simulink model "testmodel"  (R2017b)
settings: Solver=FixedStepAuto  StartTime=0.0  StopTime=inf  FixedStep=.001  RelTol=1e-3  EnableMultiTasking=on
libraries: simulink x5, dspstat3 x5
settings Model: SimulationMode=external  Creator=MRRL  LastModifiedBy=johnm_000
settings SolverCC: PositivePriorityOrder=on
settings OptimizationCC: PassReuseOutputArgsThreshold=0  MaxStackSize=64
settings DebuggingCC: ParameterTunabilityLossMsg=error
settings HardwareCC: ProdBitPerPointer=32  ProdBitPerSizeT=32  ProdBitPerPtrDiffT=32  ProdLargestAtomicInteger=Long  ProdLargestAtomicFloat=Double  ProdWordSize=32  ProdHWDeviceType=ARM Compatible->ARM Cortex  UseEmbeddedCoderFeatures=off  UseSimulinkCoderFeatures=off
settings SFSimCC: MATLABDynamicMemAlloc=off
settings RTWCC: SystemTargetFile=ert.tlc  HardwareBoard=Raspberry Pi  TemplateMakefile=ert_default_tmf  GenerateReport=on  Toolchain=GNU GCC Raspberry Pi  LaunchReport=on
settings CodeAppCC: ForceParamTrailComments=on  OperatorAnnotations=on
settings ERTTargetCC: ERTCustomFileBanners=off  SupportContinuousTime=on  SupportNonInlinedSFcns=on  RemoveResetFunc=off  SupportVariableSizeSignals=on  ModelStepFunctionPrototypeControlCompliant=off

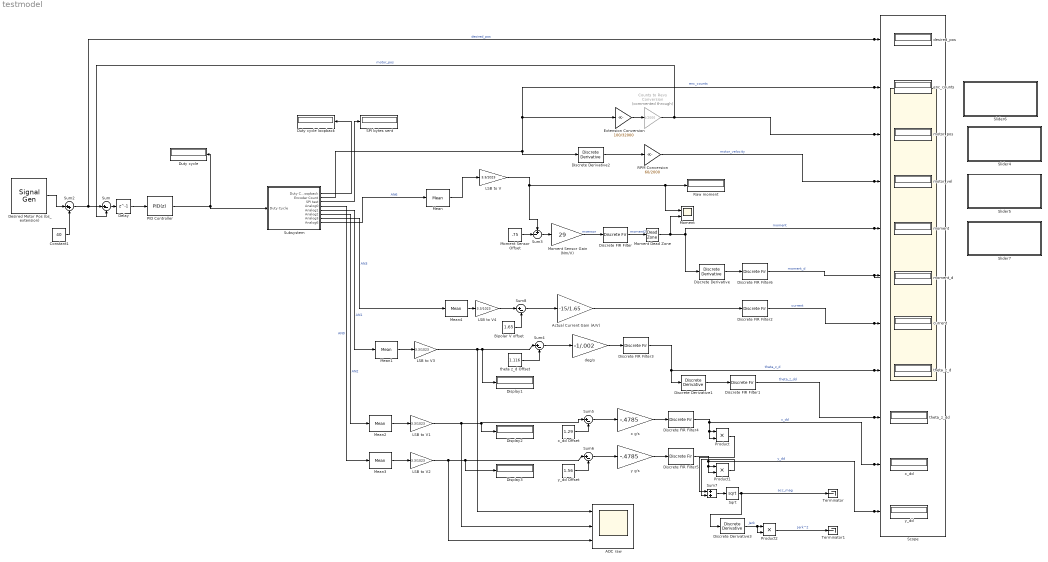
== system testmodel ==
  ADC raw : Scope  NumInputPorts=3
  Actual Current Gain (A/V) : Gain  Gain=-15/1.65
  Bipolar V offset : Constant  Value=1.65
  Constant1 : Constant  Value=40
  Counts to Revs Conversion : Gain  Commented=through  Gain=1/2000  ParamDataTypeStr=double  OutDataTypeStr=double
  Delay : Delay  DelayLength=1  InitialCondition=0
  Desired Motor Pos (bs_extension) : SignalGenerator  WaveForm=square  Amplitude=40
  Discrete Derivative{,1..3} (4 alike) : simulink/Discrete/Discrete Derivative  gainval=1.0  ICPrevScaledInput=0.0  InputProcessing=Inherited  OutMin=[]  OutMax=[]  OutDataType=fixdt(1, 16)  OutScaling=2^-10  DoSatur=off
  Discrete FIR Filter{,1..6} (7 alike) : DiscreteFir  Coefficients=[.1 .1 .1 .1 .1 .1 .1 .1 .1 .1]
  Display1 : Display
  Display2 : Display
  Display3 : Display
  Duty cycle : Display
  Duty cycle loopback : Display
  Extension Conversion : Gain  Gain=100/32000  ParamDataTypeStr=double  OutDataTypeStr=double
  LSB to V{,1..4} (5 alike) : Gain  Gain=3.3/1023
  Mean{,1..4} (5 alike) : dspstat3/Mean  run=off  reset_popup=None  InputProcessing=Columns as channels (frame based)  directionMode=Each column  dimension=1  roiEnable=off  roiType=Rectangles  roiPortion=Entire ROI  roiOutput=Individual statistics for each ROI  roiFlag=off  outputDataTypeStr=Inherit: Same as accumulator  outputLastDataTypeStr=Inherit: Same as accumulator  outputMin=[]  outputMax=[]  roundingMode=Floor  overflowMode=off
  Moment : Scope  NumInputPorts=2
  Moment Sensor Offset : Constant  Value=.75
  Moment Dead Zone : DeadZone  LowerValue=-.25  UpperValue=.25  SaturateOnIntegerOverflow=on
  Moment Sensor Gain (Nm/V) : Gain  Gain=29
  PID Controller : simulink/Continuous/PID Controller  Controller=PID  TimeDomain=Discrete-time  SampleTime=-1  IntegratorMethod=Forward Euler  FilterMethod=Forward Euler  Form=Parallel  UseFilter=on  ControllerParametersSource=internal  P=.1  I=.05  D=.003  N=300  InitialConditionSource=internal  InitialConditionForIntegrator=0  InitialConditionForFilter=0  ExternalReset=none  LimitOutput=on  UpperSaturationLimit=10  LowerSaturationLimit=-10  LinearizeAsGain=on  AntiWindupMode=none  Kb=1  TrackingMode=off  Kt=1  PParamMin=[]  PParamMax=[]  IParamMin=[]  IParamMax=[]  DParamMin=[]  DParamMax=[]  NParamMin=[]  NParamMax=[]  KbParamMin=[]  KbParamMax=[]  KtParamMin=[]  KtParamMax=[]  POutMin=[]  POutMax=[]  IOutMin=[]  IOutMax=[]  DOutMin=[]  DOutMax=[]  NOutMin=[]  NOutMax=[]  KbOutMin=[]  KbOutMax=[]  KtOutMin=[]  KtOutMax=[]  IntegratorOutMin=[]  IntegratorOutMax=[]  FilterOutMin=[]  FilterOutMax=[]  SumOutMin=[]  SumOutMax=[]  SumI1OutMin=[]  SumI1OutMax=[]  SumI2OutMin=[]  SumI2OutMax=[]  SumI3OutMin=[]  SumI3OutMax=[]  SumDOutMin=[]  SumDOutMax=[]  SaturationOutMin=[]  SaturationOutMax=[]  IntegratorContinuousStateAttributes=''  IntegratorStateMustResolveToSignalObject=off  IntegratorRTWStateStorageClass=Auto  FilterContinuousStateAttributes=''  FilterStateMustResolveToSignalObject=off  FilterRTWStateStorageClass=Auto  DifferentiatorICPrevScaledInput=0  DifferentiatorOutMin=[]  DifferentiatorOutMax=[]  InitialConditionSetting=State (most efficient)  FilterDiffOutCoefMin=[]  FilterDiffOutCoefMax=[]  SumDenOutMin=[]  SumDenOutMax=[]  SumNumOutMin=[]  SumNumOutMax=[]  ReciprocalOutMin=[]  ReciprocalOutMax=[]  DivideOutMin=[]  DivideOutMax=[]  TunerSelectOption=Transfer Function Based (PID Tuner App)
  Product : Product
  Product1 : Product
  Product2 : Product
  RPM Conversion : Gain  Gain=60/2000  ParamDataTypeStr=double  OutDataTypeStr=double
  Raw moment : Display
  SPI bytes sent : Display
  Scope : Scope  NumInputPorts=11
  Slider4 : Subsystem  DialogController=hmiCreateDDGDialog  IsWebBlock=on  mask(MWDashboardBlock){webBlockId=085e5637-d5ac-41cb-8731-7366e30fa1b6, webBlockType=slider, ShowInLibBrowser=on, ShowInitialText=on, HMISrcModelName=testmodel}
      mask prompts: webBlockId "WebBlock Id"; webBlockType "WebBlock Type"; HMISrcModelName "Source Model"
      mask Help: helpview([docroot '/mapfiles/simulink.map'], 'hmi_slider')
      mask Display:
      | if strcmp(get_param(bdroot(gcb),'BlockDiagramType'), 'library')
      |     image([(matlabroot) '/toolbox/simulink/hmi/icons/Slider.png']);
      | end
  Slider5 : Subsystem  DialogController=hmiCreateDDGDialog  IsWebBlock=on  mask(MWDashboardBlock){webBlockId=f28c714c-6520-4032-bd51-1fb2bc96d9d9, webBlockType=slider, ShowInLibBrowser=on, ShowInitialText=on, HMISrcModelName=testmodel}
      mask prompts: webBlockId "WebBlock Id"; webBlockType "WebBlock Type"; HMISrcModelName "Source Model"
      mask Help: helpview([docroot '/mapfiles/simulink.map'], 'hmi_slider')
      mask Display:
      | if strcmp(get_param(bdroot(gcb),'BlockDiagramType'), 'library')
      |     image([(matlabroot) '/toolbox/simulink/hmi/icons/Slider.png']);
      | end
  Slider6 : Subsystem  DialogController=hmiCreateDDGDialog  IsWebBlock=on  mask(MWDashboardBlock){webBlockId=46740757-b30e-4b65-9acf-b82be8f8e4ac, webBlockType=slider, ShowInLibBrowser=on, ShowInitialText=on, HMISrcModelName=testmodel}
      mask prompts: webBlockId "WebBlock Id"; webBlockType "WebBlock Type"; HMISrcModelName "Source Model"
      mask Help: helpview([docroot '/mapfiles/simulink.map'], 'hmi_slider')
      mask Display:
      | if strcmp(get_param(bdroot(gcb),'BlockDiagramType'), 'library')
      |     image([(matlabroot) '/toolbox/simulink/hmi/icons/Slider.png']);
      | end
  Slider7 : Subsystem  DialogController=hmiCreateDDGDialog  IsWebBlock=on  mask(MWDashboardBlock){webBlockId=fcfba7e5-e6d5-4b75-8ef5-2454024f1223, webBlockType=slider, ShowInLibBrowser=on, ShowInitialText=on, HMISrcModelName=testmodel}
      mask prompts: webBlockId "WebBlock Id"; webBlockType "WebBlock Type"; HMISrcModelName "Source Model"
      mask Help: helpview([docroot '/mapfiles/simulink.map'], 'hmi_slider')
      mask Display:
      | if strcmp(get_param(bdroot(gcb),'BlockDiagramType'), 'library')
      |     image([(matlabroot) '/toolbox/simulink/hmi/icons/Slider.png']);
      | end
  Sqrt : Sqrt  SaturateOnIntegerOverflow=on
  Subsystem : Subsystem
  Sum{,4..6,8} (5 alike) : Sum  Inputs=|+-
  Sum2 : Sum  Inputs=|++
  Sum3 : Sum  Inputs=+-|
  Sum7 : Sum
  Terminator : Terminator
  Terminator1 : Terminator
  current : Display
  deg/s : Gain  Gain=-1/.002
  desired_pos : Display
  enc_counts : Display
  moment : Display
  moment_d : Display
  motor_pos : Display
  motor_vel : Display
  "theta z_d Offset " : Constant  Value=1.116
  theta_z_d : Display
  theta_z_dd : Display
  x g's : Gain  Gain=-.4785
  x_dd : Display
  x_dd Offset : Constant  Value=1.29
  y g's : Gain  Gain=-.4785
  y_dd : Display
  y_dd Offset : Constant  Value=1.56
  wires:
  LSB to V4/1 -> Sum8/1
  Sum2/1 -> desired_pos/1, Scope/1, Sum/1  "desired_pos"
  Subsystem/2(Encoder Count) -> enc_counts/1, Scope/2, Extension Conversion/1, Discrete Derivative2/1  "enc_counts"
  Discrete FIR Filter6/1 -> moment_d/1, Scope/6  "moment_d"
  Extension Conversion/1 -> Counts to Revs Conversion/1
  Mean4/1 -> LSB to V4/1
  Discrete Derivative/1 -> Discrete FIR Filter6/1
  Discrete FIR Filter/1 -> Moment Dead Zone/1  "moment2"
  PID Controller/1 -> Subsystem/1(Duty Cycle), Duty cycle/1
  Subsystem/7(Analog3) -> Mean4/1  "AN3"
  LSB to V1/1 -> ADC raw/2, Display2/1, Sum5/1
  Subsystem/4(Analog0) -> Mean3/1  "AN0"
  Desired Motor Pos (bs_extension)/1 -> Sum2/1
  x_dd Offset/1 -> Sum5/2
  Counts to Revs Conversion/1 -> motor_pos/1, Scope/3, Sum/2  "motor_pos"
  Constant1/1 -> Sum2/2
  Subsystem/3(SPI test) -> SPI bytes sent/1
  RPM Conversion/1 -> motor_vel/1, Scope/4  "motor_velocity"
  Mean3/1 -> LSB to V2/1
  Bipolar V offset/1 -> Sum8/2
  LSB to V/1 -> Sum3/1, Raw moment/1, Moment/1
  Moment Dead Zone/1 -> moment/1, Scope/5, Discrete Derivative/1, Moment/2  "moment"
  Sum7/1 -> Sqrt/1
  Mean/1 -> LSB to V/1
  Product/1 -> Sum7/1
  Moment Sensor Offset/1 -> Sum3/2
  Discrete Derivative2/1 -> RPM Conversion/1
  Product1/1 -> Sum7/2
  Product2/1 -> Terminator1/1  "Jerk^2"
  Discrete FIR Filter5/1 -> y_dd/1, Scope/11, Product1/2, Product1/1  "y_dd"
  Moment Sensor Gain (Nm/V)/1 -> Discrete FIR Filter/1  "msensor"
  x g's/1 -> Discrete FIR Filter4/1
  Discrete FIR Filter4/1 -> x_dd/1, Scope/10, Product/2, Product/1  "x_dd"
  Actual Current Gain (A/V)/1 -> Discrete FIR Filter2/1
  y g's/1 -> Discrete FIR Filter5/1
  Discrete Derivative3/1 -> Product2/2, Product2/1  "Jerk"
  Sum6/1 -> y g's/1
  Subsystem/1(Duty Cycle Loopback) -> Duty cycle loopback/1
  Subsystem/8(Analog6) -> Mean/1  "AN6"
  y_dd Offset/1 -> Sum6/2
  Discrete FIR Filter1/1 -> theta_z_dd/1, Scope/9  "theta_z_dd"
  Mean1/1 -> LSB to V3/1
  Sqrt/1 -> Terminator/1, Discrete Derivative3/1  "acc_mag"
  Sum8/1 -> Actual Current Gain (A/V)/1
  LSB to V2/1 -> ADC raw/3, Display3/1, Sum6/1
  Sum5/1 -> x g's/1
  "theta z_d Offset "/1 -> Sum4/2
  Subsystem/5(Analog1) -> Mean1/1  "AN1"
  Delay/1 -> PID Controller/1
  LSB to V3/1 -> ADC raw/1, Display1/1, Sum4/1
  Subsystem/6(Analog2) -> Mean2/1  "AN2"
  Sum4/1 -> deg/s/1
  Discrete FIR Filter3/1 -> theta_z_d/1, Scope/8, Discrete Derivative1/1  "theta_z_d"
  Sum3/1 -> Moment Sensor Gain (Nm/V)/1
  Discrete FIR Filter2/1 -> current/1, Scope/7  "current"
  Discrete Derivative1/1 -> Discrete FIR Filter1/1
  Sum/1 -> Delay/1
  deg/s/1 -> Discrete FIR Filter3/1
  Mean2/1 -> LSB to V1/1

== system testmodel/Slider4 ==

== system testmodel/Slider5 ==

== system testmodel/Slider6 ==

== system testmodel/Slider7 ==

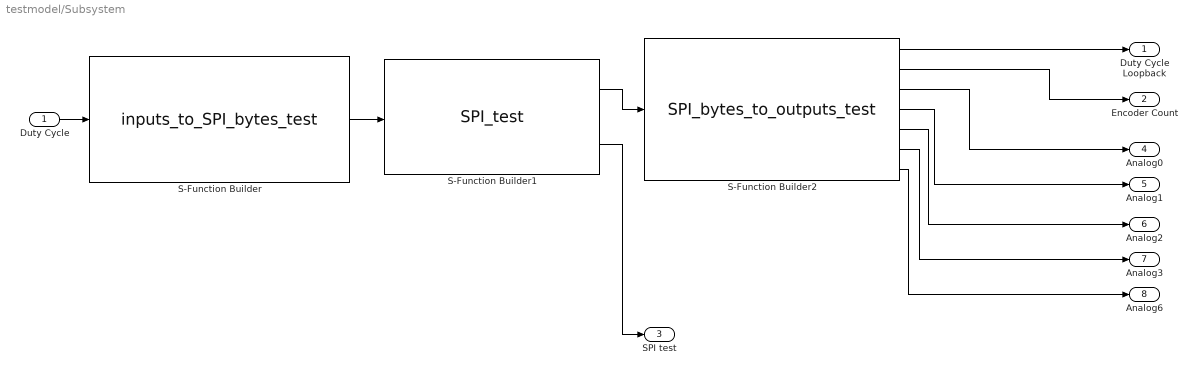
== system testmodel/Subsystem ==
  Duty Cycle : Inport
  S-Function Builder : S-Function  InitFcn=try, set_param(gcb,'FunctionName','inputs_to_SPI_bytes_test'), end  FunctionName=inputs_to_SPI_bytes_test  SFunctionModules=inputs_to_SPI_bytes_test_wrapper  SFunctionDeploymentMode=off  EnableBusSupport=off  mask(S-Function Builder){}
      mask help: Simulink:masks:SFunctionBuilder_MD
      mask init:
      | val = [[.9  0.75 0.75 1 1 .9 .9 1]',[1 1 0.75 0.75 .9 .9 1 .9]'];try , sys = get_param(gcb,'SfunBuilderFcnName');if isempty(sys), sys = get_param(gcb,'FunctionName'); end,catch, sys = get_param(gcb,'FunctionName'); end
      settings: CopyFcn=set_param(gcbh,'LinkStatus','none')  PreSaveFcn=try, set_param(gcb,'FunctionName','inputs_to_SPI_bytes_test'), end  OpenFcn=sfunctionwizard(gcbh)
      mask Display: plot(val(:,1),val(:,2)),disp(sys), port_label('input',1,'dutyCycle'), port_label('output',1,'write')
  S-Function Builder1 : S-Function  InitFcn=try, set_param(gcb,'FunctionName','SPI_test'), end  FunctionName=SPI_test  SFunctionModules=SPI_test_wrapper  SFunctionDeploymentMode=off  EnableBusSupport=off  mask(S-Function Builder){}
      mask help: Simulink:masks:SFunctionBuilder_MD
      mask init: same as testmodel/Subsystem/S-Function Builder
      settings: CopyFcn=set_param(gcbh,'LinkStatus','none')  PreSaveFcn=try, set_param(gcb,'FunctionName','SPI_test'), end  OpenFcn=sfunctionwizard(gcbh)
      mask Display: plot(val(:,1),val(:,2)),disp(sys), port_label('input',1,'write'), port_label('output',1,'read'), port_label('output',2,'spi_test')
  S-Function Builder2 : S-Function  InitFcn=try, set_param(gcb,'FunctionName','SPI_bytes_to_outputs_test'), end  FunctionName=SPI_bytes_to_outputs_test  SFunctionModules=SPI_bytes_to_outputs_test_wrapper  SFunctionDeploymentMode=off  EnableBusSupport=off  mask(S-Function Builder){}
      mask help: Simulink:masks:SFunctionBuilder_MD
      mask init: same as testmodel/Subsystem/S-Function Builder
      settings: CopyFcn=set_param(gcbh,'LinkStatus','none')  PreSaveFcn=try, set_param(gcb,'FunctionName','SPI_bytes_to_outputs_test'), end  OpenFcn=sfunctionwizard(gcbh)
      mask Display: plot(val(:,1),val(:,2)),disp(sys), port_label('input',1,'read'), port_label('output',1,'dutyCycle'), port_label('output',2,'enc1count'), port_label('output',3,'analog0'), port_label('output',4,'analog1'), port_label('output',5,'analog2'), port_label('output',6,'analog3'), port_label('output',7,'analog6')
  Duty Cycle Loopback : Outport
  Encoder Count : Outport  Port=2
  SPI test : Outport  Port=3
  Analog0 : Outport  Port=4
  Analog1 : Outport  Port=5
  Analog2 : Outport  Port=6
  Analog3 : Outport  Port=7
  Analog6 : Outport  Port=8
  wires:
  Duty Cycle/1 -> S-Function Builder/1
  S-Function Builder/1 -> S-Function Builder1/1
  S-Function Builder1/2 -> SPI test/1
  S-Function Builder1/1 -> S-Function Builder2/1
  S-Function Builder2/1 -> Duty Cycle Loopback/1
  S-Function Builder2/2 -> Encoder Count/1
  S-Function Builder2/3 -> Analog0/1
  S-Function Builder2/4 -> Analog1/1
  S-Function Builder2/5 -> Analog2/1
  S-Function Builder2/6 -> Analog3/1
  S-Function Builder2/7 -> Analog6/1
